simulink model "NEW_B747_lateral_per"  (R2016b)
settings: Solver=ode45  StartTime=0.0  StopTime=150  RelTol=1e-3  EnableMultiTasking=on
values from neighbouring files (symbols this model uses):
  A_per = [Yb(FLIGHT_CONDITION_PER)/U_per 0 -1 g/U_per*cos(gamma0) 0 ... (first row only)    [lateral.m]
  B_per = [0 Ydr(FLIGHT_CONDITION_PER) ... (first row only)    [lateral.m]
  Bex_per = [Bex_per B_per]    [lateral.m]
  C = [0 1 0 0 0 ... (first row only)    [lateral.m]
  K = M1/X11    [lateral.m]
  L = X21\Z1    [lateral.m]
  U_per = a(FLIGHT_CONDITION_PER)*M(FLIGHT_CONDITION_PER)    [lateral.m]
undefined symbols (not defined in the file or in its folder): denHp_per, denHr_per, denHv_per, numHp_per, numHr_per, numHv_per
libraries: simulink_extras x11, simulink x2
settings Model: Creator=Ivan  LastModifiedBy=ivan
settings DataIOCC: LimitDataPoints=on  SaveFormat=Array
settings OptimizationCC: LifeSpan=inf
settings DebuggingCC: AllowSymbolicDim=off  SFUnexpectedBacktrackingDiag=warning  SFNoUnconditionalDefaultTransitionDiag=warning  SFExecutionAtInitializationDiag=none
settings HardwareCC: ProdBitPerPointer=32  ProdBitPerSizeT=32  ProdBitPerPtrDiffT=32  ProdLargestAtomicFloat=None  ProdIntDivRoundTo=Undefined  ProdEndianess=Unspecified  ProdWordSize=32  ProdHWDeviceType=32-bit Generic
settings ModelReferenceCC: PropagateSignalLabelsOutOfModel=off
settings GRTTargetCC: TargetLangStandard=C89/C90 (ANSI)  GeneratePreprocessorConditionals=Disable all
settings ConfigComp: CovMetricSettings=dw  CovHtmlReporting=on  CovSaveCumulativeToWorkspaceVar=on  CovSaveSingleToWorkspaceVar=on  CovExternalEMLEnable=off

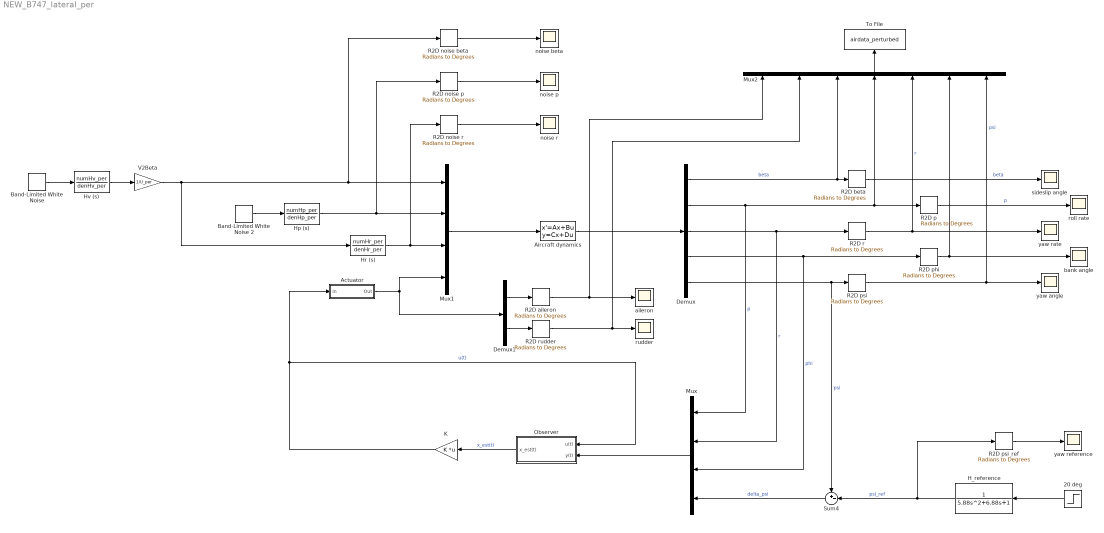
== system NEW_B747_lateral_per ==
  20 deg : Step  Time=0  After=20*pi/180
  Actuator : Subsystem
  Aircraft dynamics : StateSpace  A=A_per  B=Bex_per  C=eye(5)  D=zeros(5,5)  X0=0
  Band-Limited White Noise : simulink/Sources/Band-Limited White Noise  Cov=[0.001]  Ts=0.02  seed=[23341]
  Band-Limited White Noise 2 : simulink/Sources/Band-Limited White Noise  Cov=[0.01]  Ts=0.02  seed=[23341]
  Demux : Demux  Outputs=5
  Demux1 : Demux  Outputs=2
  H_reference : TransferFcn  Denominator=[5.88 6.88 1]
  Hp (s) : TransferFcn  Numerator=numHp_per  Denominator=denHp_per
  Hr (s) : TransferFcn  Numerator=numHr_per  Denominator=denHr_per
  Hv (s) : TransferFcn  Numerator=numHv_per  Denominator=denHv_per
  K : Gain  Gain=K  Multiplication=Matrix(K*u)
  Mux : Mux
  Mux1 : Mux  Inputs=[1 1 1 2]
  Mux2 : Mux  Inputs=7
  Observer : Subsystem
  R2D aileron : simulink_extras/Transformations/Radians to Degrees
  R2D beta : simulink_extras/Transformations/Radians to Degrees
  R2D noise beta : simulink_extras/Transformations/Radians to Degrees
  R2D noise p : simulink_extras/Transformations/Radians to Degrees
  R2D noise r : simulink_extras/Transformations/Radians to Degrees
  R2D p : simulink_extras/Transformations/Radians to Degrees
  R2D phi : simulink_extras/Transformations/Radians to Degrees
  R2D psi : simulink_extras/Transformations/Radians to Degrees
  R2D psi_ref : simulink_extras/Transformations/Radians to Degrees
  R2D r : simulink_extras/Transformations/Radians to Degrees
  R2D rudder : simulink_extras/Transformations/Radians to Degrees
  Sum4 : Sum  Inputs=+-|
  To File : ToFile  Filename=airdata_perturbed  MatrixName=out_per  SaveFormat=Timeseries
  V2Beta : Gain  Gain=1/U_per
  aileron : Scope
  bank angle : Scope
  noise beta : Scope
  noise p : Scope
  noise r : Scope
  roll rate : Scope
  rudder : Scope
  sideslip angle : Scope
  yaw angle : Scope
  yaw rate : Scope
  yaw reference : Scope
  wires:
  K/1 -> Observer/1(u(t)), Actuator/1(In)  "u(t)"
  Aircraft dynamics/1 -> Demux/1
  R2D beta/1 -> sideslip angle/1  "beta"
  Mux/1 -> Observer/2(y(t))
  Observer/1(x_est(t)) -> K/1  "x_est(t)"
  20 deg/1 -> H_reference/1
  Demux/1 -> Mux2/3, R2D beta/1  "beta"
  Demux/2 -> Mux/1, R2D p/1, Mux2/4  "p"
  R2D p/1 -> roll rate/1  "p"
  Demux/3 -> Mux/2, R2D r/1  "r"
  R2D r/1 -> Mux2/5, yaw rate/1  "r"
  Demux/4 -> R2D phi/1, Mux/3  "phi"
  R2D phi/1 -> Mux2/6, bank angle/1
  Demux/5 -> R2D psi/1, Sum4/1  "psi"
  R2D psi/1 -> yaw angle/1, Mux2/7  "psi"
  Sum4/1 -> Mux/4  "delta_psi"
  H_reference/1 -> Sum4/2, R2D psi_ref/1  "psi_ref"
  R2D rudder/1 -> Mux2/2, rudder/1
  R2D aileron/1 -> Mux2/1, aileron/1
  Demux1/1 -> R2D aileron/1
  Demux1/2 -> R2D rudder/1
  Actuator/1(Out) -> Demux1/1, Mux1/4
  R2D psi_ref/1 -> yaw reference/1
  Mux2/1 -> To File/1
  Band-Limited White Noise/1 -> Hv (s)/1
  Hv (s)/1 -> V2Beta/1
  Band-Limited White Noise 2/1 -> Hp (s)/1
  Hp (s)/1 -> Mux1/2, R2D noise p/1
  Hr (s)/1 -> Mux1/3, R2D noise r/1
  V2Beta/1 -> Hr (s)/1, Mux1/1, R2D noise beta/1
  R2D noise p/1 -> noise p/1
  R2D noise r/1 -> noise r/1
  R2D noise beta/1 -> noise beta/1
  Mux1/1 -> Aircraft dynamics/1

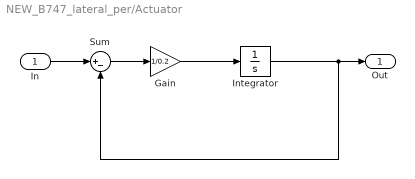
== system NEW_B747_lateral_per/Actuator ==
  In : Inport
  Gain : Gain  Gain=1/0.2
  Integrator : Integrator
  Sum : Sum  Inputs=|+-
  Out : Outport
  wires:
  In/1 -> Sum/1
  Gain/1 -> Integrator/1
  Integrator/1 -> Sum/2, Out/1
  Sum/1 -> Gain/1

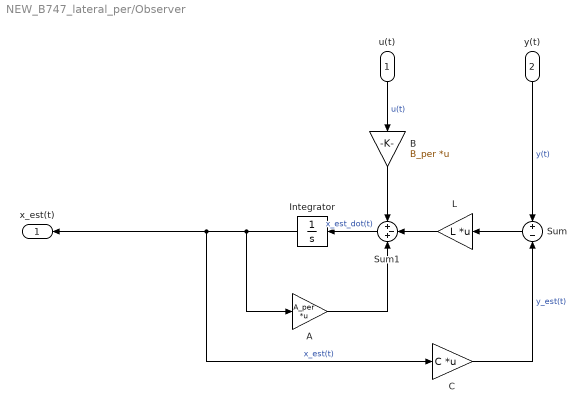
== system NEW_B747_lateral_per/Observer ==
  u(t) : Inport
  y(t) : Inport  Port=2
  A : Gain  Gain=A_per  Multiplication=Matrix(K*u)
  B : Gain  Gain=B_per  Multiplication=Matrix(K*u)
  C : Gain  Gain=C  Multiplication=Matrix(K*u)
  Integrator : Integrator
  L : Gain  Gain=L  Multiplication=Matrix(K*u)
  Sum : Sum  Inputs=+-
  Sum1 : Sum  Inputs=+-+
  x_est(t) : Outport
  wires:
  u(t)/1 -> B/1  "u(t)"
  L/1 -> Sum1/2
  Sum1/1 -> Integrator/1  "x_est_dot(t)"
  Integrator/1 -> x_est(t)/1, C/1, A/1  "x_est(t)"
  A/1 -> Sum1/3
  B/1 -> Sum1/1
  Sum/1 -> L/1
  C/1 -> Sum/2  "y_est(t)"
  y(t)/1 -> Sum/1  "y(t)"
